simulink model "UE_Simulator"  (R2021b)
settings: Solver=ode4  StartTime=0.0  StopTime=100.0  FixedStep=0.1  RelTol=1e-3
settings Model: Creator=Mario  LastModifiedBy=Mario

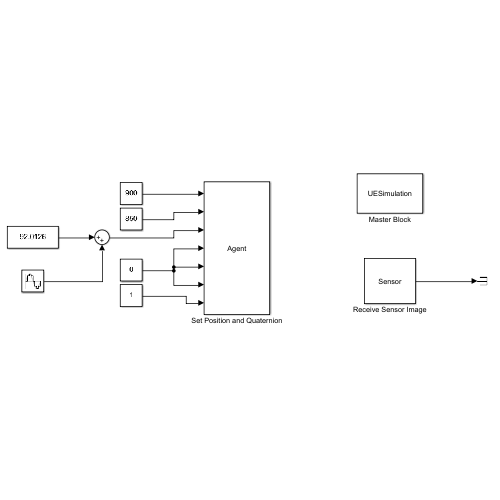
[thumbnail: Simulink's stored preview of the top-level diagram]
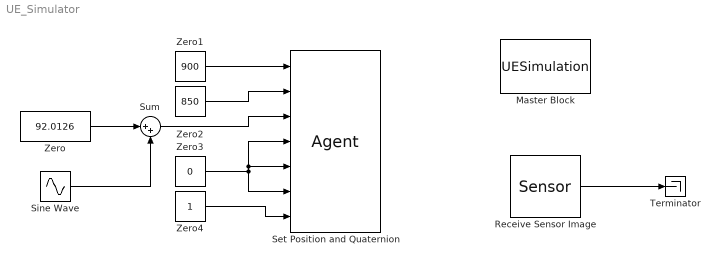
== system UE_Simulator ==
  Master Block : M-S-Function  Priority=0  FunctionName=UESimulation
  Receive Sensor Image : M-S-Function  Priority=1  FunctionName=Sensor
  Set Position and Quaternion : M-S-Function  Priority=-1  FunctionName=Agent
  Sine Wave : Sin  Amplitude=100  Bias=600  Frequency=2*pi*1  SampleTime=0.1
  Sum : Sum  Inputs=|++
  Terminator : Terminator
  Zero : Constant  Value=92.0126  OutDataTypeStr=double
  Zero1 : Constant  Value=900  OutDataTypeStr=double
  Zero2 : Constant  Value=850  OutDataTypeStr=double
  Zero3 : Constant  Value=0  OutDataTypeStr=double
  Zero4 : Constant  OutDataTypeStr=double
  wires:
  Zero1/1 -> Set Position and Quaternion/1
  Zero2/1 -> Set Position and Quaternion/2
  Zero3/1 -> Set Position and Quaternion/6, Set Position and Quaternion/5, Set Position and Quaternion/4
  Zero4/1 -> Set Position and Quaternion/7
  Zero/1 -> Sum/1
  Sine Wave/1 -> Sum/2
  Sum/1 -> Set Position and Quaternion/3
  Receive Sensor Image/1 -> Terminator/1
